simulink model "rodaReacaoCaracteristicas"  (R2024a)
settings: Solver=FixedStepAuto  StartTime=0.0  StopTime=tf  FixedStep=step_modelo  RelTol=1e-3
values from neighbouring files (symbols this model uses):
  B = norm(B_vec)    [orb_elem.m]
undefined symbols (not defined in the file or in its folder): Iw, Ixx, Iyy, Izz, Km, Kv, limCorrente, limVolt, Rm, RodKi, RotMax, TdRod, Tmax, TpulseRod
settings Model: PacingRate=1000  VariantFading=off  Creator=rodri  LastModifiedBy=rodri
settings DataIOCC: SaveOutput=off  SaveTime=off
settings RTWCC: GPUComputeCapability=3.5

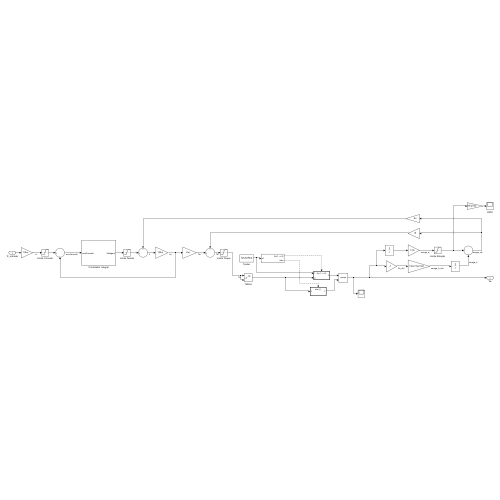
[thumbnail: Simulink's stored preview of the top-level diagram]
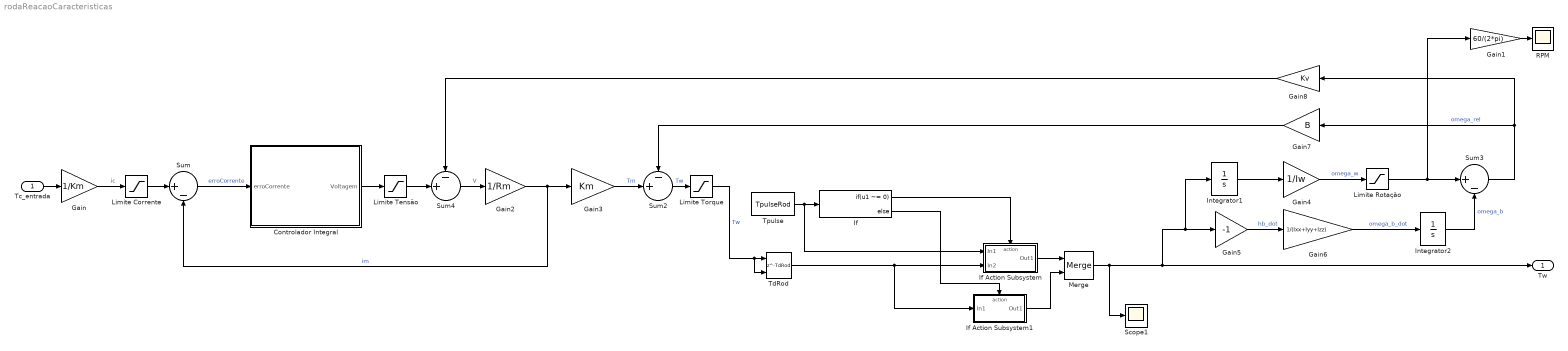
== system rodaReacaoCaracteristicas ==
  Tc_entrada : Inport  OutDataTypeStr=double  PortDimensions=1  SampleTime=0
  Controlador Integral : Subsystem
  Gain : Gain  Gain=1/Km
  Gain1 : Gain  Gain=60/(2*pi)
  Gain2 : Gain  Gain=1/Rm
  Gain3 : Gain  Gain=Km
  Gain4 : Gain  Gain=1/Iw
  Gain5 : Gain  Gain=-1
  Gain6 : Gain  Gain=1/(Ixx+Iyy+Izz)
  Gain7 : Gain  Gain=B
  Gain8 : Gain  Gain=Kv
  If : If  IfExpression=u1 ~= 0
  If Action Subsystem : Subsystem  TreatAsAtomicUnit=on
  If Action Subsystem1 : Subsystem  TreatAsAtomicUnit=on
  Integrator1 : Integrator
  Integrator2 : Integrator
  Limite Corrente : Saturate  UpperLimit=limCorrente  LowerLimit=-limCorrente
  Limite Rotação : Saturate  UpperLimit=RotMax*2*pi/60  LowerLimit=-RotMax*2*pi/60
  Limite Tensão : Saturate  UpperLimit=limVolt  LowerLimit=-limVolt
  Limite Torque : Saturate  UpperLimit=Tmax  LowerLimit=-Tmax
  Merge : Merge
  RPM : Scope
  Scope1 : Scope
  Sum : Sum  Inputs=|+-
  Sum2 : Sum  Inputs=-+|
  Sum3 : Sum  Inputs=|+-
  Sum4 : Sum  Inputs=-+|
  TdRod : Delay  DelayLength=TdRod  InitialConditionSource=Input port  InitialCondition=0
      settings: InputPortMap=u0,p4
  Tpulse : Constant  Value=TpulseRod  SampleTime=-1
  Tw : Outport  OutDataTypeStr=double  PortDimensions=1  SampleTime=0
  wires:
  Sum3/1 -> Gain8/1, Gain7/1  "omega_rel"
  Integrator2/1 -> Sum3/2  "omega_b"
  Gain2/1 -> Sum/2, Gain3/1  "im"
  Sum4/1 -> Gain2/1  "V"
  Integrator1/1 -> Gain4/1
  Gain3/1 -> Sum2/2  "Tm"
  Limite Torque/1 -> TdRod/1, TdRod/2  "Tw"
  Gain7/1 -> Sum2/1
  Limite Corrente/1 -> Sum/1
  Tc_entrada/1 -> Gain/1
  Gain/1 -> Limite Corrente/1  "ic"
  Controlador Integral/1(Voltagem) -> Limite Tensão/1
  Gain8/1 -> Sum4/1
  Gain6/1 -> Integrator2/1  "omega_b_dot"
  Gain5/1 -> Gain6/1  "hb_dot"
  Sum/1 -> Controlador Integral/1(erroCorrente)  "erroCorrente"
  Limite Tensão/1 -> Sum4/2
  Gain1/1 -> RPM/1
  Gain4/1 -> Limite Rotação/1  "omega_w"
  Limite Rotação/1 -> Gain1/1, Sum3/1
  Sum2/1 -> Limite Torque/1  "Tw"
  Tpulse/1 -> If Action Subsystem/1(In1), If/1
  If Action Subsystem/1(Out1) -> Merge/1
  If Action Subsystem1/1(Out1) -> Merge/2
  If/2 -> If Action Subsystem1/Action
  If/1 -> If Action Subsystem/Action
  Merge/1 -> Tw/1, Gain5/1, Integrator1/1, Scope1/1
  TdRod/1 -> If Action Subsystem1/1(In1), If Action Subsystem/2(In2)

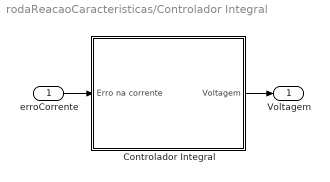
== system rodaReacaoCaracteristicas/Controlador Integral ==
  erroCorrente : Inport
  Controlador Integral : Subsystem
  Voltagem : Outport
  wires:
  erroCorrente/1 -> Controlador Integral/1(Erro na corrente)
  Controlador Integral/1(Voltagem) -> Voltagem/1

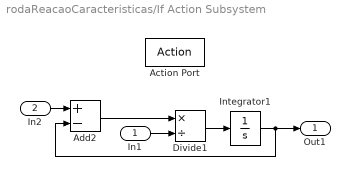
== system rodaReacaoCaracteristicas/If Action Subsystem ==
  In1 : Inport
  In2 : Inport  Port=2
  Action Port : ActionPort  ActionPortLabel=if(u1 ~= 0)
  Add2 : Sum  Inputs=+-
  Divide1 : Product  Inputs=*/
  Integrator1 : Integrator
  Out1 : Outport
  wires:
  In2/1 -> Add2/1
  Integrator1/1 -> Out1/1, Add2/2
  Add2/1 -> Divide1/1
  Divide1/1 -> Integrator1/1
  In1/1 -> Divide1/2

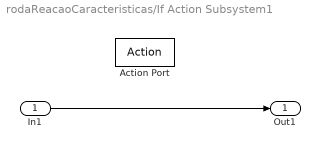
== system rodaReacaoCaracteristicas/If Action Subsystem1 ==
  In1 : Inport
  Action Port : ActionPort  ActionPortLabel=else
  Out1 : Outport
  wires:
  In1/1 -> Out1/1

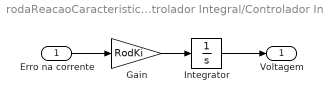
== system rodaReacaoCaracteristicas/Controlador Integral/Controlador Integral ==
  Erro na corrente : Inport
  Gain : Gain  Gain=RodKi
  Integrator : Integrator
  Voltagem : Outport  VectorParamsAs1DForOutWhenUnconnected=off
  wires:
  Integrator/1 -> Voltagem/1
  Erro na corrente/1 -> Gain/1
  Gain/1 -> Integrator/1
